simulink model "timeds_m"  (Simulink 7.9)
settings: Solver=ode45  SolverMode=SingleTasking  StartTime=0.0  StopTime=999999  MaxStep=10  RelTol=1e-3  AbsTol=1e-3
values from neighbouring files (symbols this model uses):
  U = st_Varia('LongNames')    [timeds_i.m]
  x0 = zeros(P.NumCel,1)    [timeds_i.m]    (also in timeds_s.m = x0)
undefined symbols (not defined in the file or in its folder): B
settings Model: Creator=M.Sparnaaij  LastModifiedBy=M.Sparnaaij
settings DataIOCC: LimitDataPoints=off  SaveOutput=off  SaveTime=off  SignalLoggingName=sigsOut
settings OptimizationCC: BooleanDataType=off
settings DebuggingCC: SaveWithParameterizedLinksMsg=none  SignalResolutionControl=TryResolveAllWithWarning  SolverPrmCheckMsg=none  MultiTaskDSMMsg=warning  MultiTaskCondExecSysMsg=none  StrictBusMsg=None
settings HardwareCC: TargetUnknown=on
settings RTWCC: IncludeERTFirstTime=on
settings GRTTargetCC: CombineOutputUpdateFcns=off  GRTInterface=on

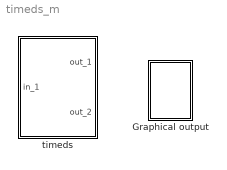
== system timeds_m ==
  Graphical output : Subsystem
      settings: OpenFcn=timeds_g
      mask Display:
      | plot(0,0,100,100,[80,20,20],[20,20,80],[80,69,60,52,45,39,33,28,24,20],[65,65,64,61,57,52,45,37,30,20])
      | disp('');
      | text(100,100,'timeds', 'horizontalAlignment', 'right', 'verticalAlignment', 'top');
  timeds : Subsystem  Description=This model calculates the removal of suspended solids with a single media filter.
      mask init:
      | filenaam='.\StimelaData\Time_distribution_TD.mat';
      | 
      | [Pn,Fn,Fext]=Fileprop(filenaam);
      | 
      | errstr = st_UniqName(filenaam,'filenaam=''','SubSystem','OpenFcn');
      | if errstr, error([errstr 'The filename "' filenaam '" is already in use. Choose a different filename.']), end
      | 
      | P = timeds_p(filenaam);
      | [B,x0,U]=timeds_i(filenaam);
      settings: OpenFcn=|
      | filenaam='.\StimelaData\Time_distribution_TD.mat';
      | st_ParameterInput('init',gcb,filenaam,'timeds');
      mask Display:
      | plot(0,0,100,100,[80,20,20],[20,20,80],[80,70,65,60,55,50,45,40,35,30,20],[20,24,32,50,60,64,60,50,32,24,20])
      | disp('')
      | text(50,50,'timeds', 'horizontalAlignment', 'center', 'verticalAlignment', 'middle');
      | text(50,0,Fn, 'horizontalAlignment', 'center', 'verticalAlignment', 'base');

== system timeds_m/Graphical output ==
  note: plotten

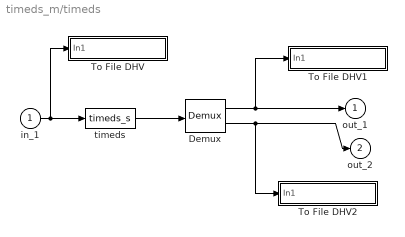
== system timeds_m/timeds ==
  in_1 : Inport
  Demux : Demux  Outputs=[U.Number B.Measurements]
  To File DHV : Subsystem  mask(To File DHV){naam=[filenaam(1:length(filenaam)-4) '_in.sti']}
      mask prompts: naam "Naam van bestand"
      mask init:
      | set_param([gcb '/To File'],'Filename',naam);
      mask Display: disp(naam)
  To File DHV1 : Subsystem  mask(To File DHV){naam=[filenaam(1:length(filenaam)-4) '_out.sti']}
      mask prompts: naam "Naam van bestand"
      mask init:
      | set_param([gcb '/To File'],'Filename',naam);
      mask Display: disp(naam)
  To File DHV2 : Subsystem  mask(To File DHV){naam=[filenaam(1:length(filenaam)-4) '_EM.sti']}
      mask prompts: naam "Naam van bestand"
      mask init:
      | set_param([gcb '/To File'],'Filename',naam);
      mask Display: disp(naam)
  timeds : S-Function  FunctionName=timeds_s  Parameters=B,x0,U,P  EnableBusSupport=off
  out_1 : Outport  InitialOutput=0
  out_2 : Outport  Port=2  InitialOutput=0
  wires:
  in_1/1 -> To File DHV/1(In1), timeds/1
  Demux/2 -> To File DHV2/1(In1), out_2/1
  Demux/1 -> To File DHV1/1(In1), out_1/1
  timeds/1 -> Demux/1

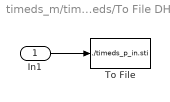
== system timeds_m/timeds/To File DHV ==
  In1 : Inport
  To File : ToFile  Filename=./timeds_p_in.sti  MatrixName=timedsin
  wires:
  In1/1 -> To File/1

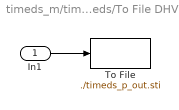
== system timeds_m/timeds/To File DHV1 ==
  In1 : Inport
  To File : ToFile  Filename=./timeds_p_out.sti  MatrixName=timedsout
  wires:
  In1/1 -> To File/1

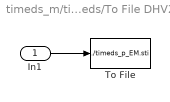
== system timeds_m/timeds/To File DHV2 ==
  In1 : Inport
  To File : ToFile  Filename=./timeds_p_EM.sti  MatrixName=timedsEM
  wires:
  In1/1 -> To File/1
